simulink library "fsw_lib"  (R2016b)
settings: Solver=VariableStepAuto  StartTime=0.0  StopTime=10.0  RelTol=1e-3
libraries: actuator_processing x1, attitude_estimation_lib x1, command_generation x1, env_estimation_lib x1, mode_selection x1, target_generation_lib x1, telemetry x1
settings Model: Creator=taylorreynolds  LastModifiedBy=Taylor

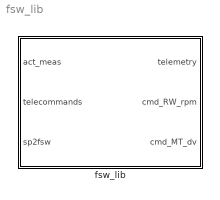
== system fsw_lib ==
  fsw_lib : Subsystem

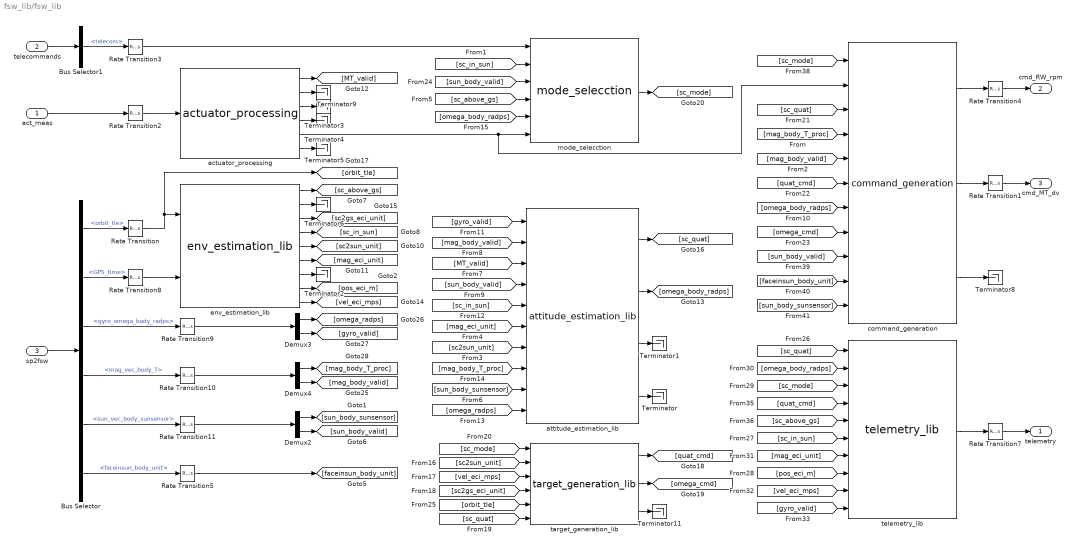
== system fsw_lib/fsw_lib ==
  act_meas : Inport
  telecommands : Inport  Port=2  OutDataTypeStr=Bus: telecommands
  sp2fsw : Inport  Port=3  OutDataTypeStr=Bus: sp2fsw
  Bus Selector : BusSelector  OutputSignals=orbit_tle,GPS_time,gyro_omega_body_radps,mag_vec_body_T,sun_vec_body_sunsensor,faceinsun_body_unit
  Bus Selector1 : BusSelector  OutputSignals=telecom
  Demux2 : Demux  Outputs=[3 1]
  Demux3 : Demux  Outputs=[3 1]
  Demux4 : Demux  Outputs=[3 1]
  Rate Transition : RateTransition  X0=fsw_params.env_estimation.ic.orbit_tle  OutPortSampleTime=fsw_params.sample_time_s
  Rate Transition1 : RateTransition
  Rate Transition{2..3,5,9..11} (6 alike) : RateTransition  OutPortSampleTime=fsw_params.sample_time_s
  Rate Transition4 : RateTransition
  Rate Transition7 : RateTransition
  Rate Transition8 : RateTransition  X0=fsw_params.sensor_processing.gps.ic.time  OutPortSampleTime=fsw_params.sample_time_s
  Terminator{,1..6,8..9,11} (10 alike) : Terminator
  actuator_processing : actuator_processing/actuator_processing
  attitude_estimation_lib : attitude_estimation_lib/attitude_estimation_lib
  command_generation : command_generation/command_generation
  env_estimation_lib : env_estimation_lib/env_estimation_lib
  mode_selecction : mode_selection/mode_selecction
  target_generation_lib : target_generation_lib/target_generation_lib
  telemetry_lib : telemetry/telemetry_lib
  "telemetry " : Outport
  cmd_RW_rpm : Outport  Port=2
  cmd_MT_dv : Outport  Port=3
  wires:
  [sc_above_gs] -> telemetry_lib/5
  Rate Transition5/1 -> [faceinsun_body_unit]
  Bus Selector/6 -> Rate Transition5/1  "<faceinsun_body_unit>"
  [sun_body_valid] -> mode_selecction/3
  [sc_above_gs] -> mode_selecction/4
  [omega_body_radps] -> mode_selecction/5
  actuator_processing/6 -> Terminator5/1
  Rate Transition4/1 -> cmd_RW_rpm/1
  Rate Transition1/1 -> cmd_MT_dv/1
  env_estimation_lib/8 -> [pos_eci_m]
  env_estimation_lib/9 -> [vel_eci_mps]
  [pos_eci_m] -> telemetry_lib/8
  [gyro_valid] -> telemetry_lib/10
  [vel_eci_mps] -> telemetry_lib/9
  [mag_eci_unit] -> telemetry_lib/7
  [sc_in_sun] -> telemetry_lib/6
  [quat_cmd] -> telemetry_lib/4
  [sc_mode] -> telemetry_lib/3
  [omega_body_radps] -> telemetry_lib/2
  [sc_quat] -> telemetry_lib/1
  Rate Transition9/1 -> Demux3/1
  Rate Transition10/1 -> Demux4/1
  Demux4/2 -> [mag_body_valid]
  Demux4/1 -> [mag_body_T_proc]
  Demux3/2 -> [gyro_valid]
  Demux3/1 -> [omega_radps]
  command_generation/2 -> Rate Transition1/1
  [sc_mode] -> command_generation/1
  [sc_mode] -> target_generation_lib/1
  mode_selecction/1 -> [sc_mode]
  target_generation_lib/3 -> Terminator11/1
  Rate Transition3/1 -> mode_selecction/1
  Rate Transition7/1 -> "telemetry "/1
  telecommands/1 -> Bus Selector1/1
  Rate Transition2/1 -> actuator_processing/1
  sp2fsw/1 -> Bus Selector/1
  telemetry_lib/1 -> Rate Transition7/1
  target_generation_lib/2 -> [omega_cmd]
  target_generation_lib/1 -> [quat_cmd]
  [orbit_tle] -> target_generation_lib/5
  [sc_quat] -> target_generation_lib/6
  [sc2gs_eci_unit] -> target_generation_lib/4
  [vel_eci_mps] -> target_generation_lib/3
  [sc2sun_unit] -> target_generation_lib/2
  actuator_processing/5 -> mode_selecction/6, command_generation/2
  attitude_estimation_lib/2 -> [omega_body_radps]
  Bus Selector/2 -> Rate Transition8/1  "<GPS_time>"
  actuator_processing/2 -> Terminator9/1
  actuator_processing/1 -> [MT_valid]
  act_meas/1 -> Rate Transition2/1
  Demux2/2 -> [sun_body_valid]
  Demux2/1 -> [sun_body_sunsensor]
  Bus Selector/5 -> Rate Transition11/1  "<sun_vec_body_sunsensor>"
  Bus Selector/4 -> Rate Transition10/1  "<mag_vec_body_T>"
  Bus Selector/3 -> Rate Transition9/1  "<gyro_omega_body_radps>"
  [sc_in_sun] -> mode_selecction/2
  [mag_body_valid] -> attitude_estimation_lib/2
  [gyro_valid] -> attitude_estimation_lib/1
  env_estimation_lib/4 -> [sc_in_sun]
  [MT_valid] -> attitude_estimation_lib/3
  [sun_body_valid] -> attitude_estimation_lib/4
  [sc_in_sun] -> attitude_estimation_lib/5
  attitude_estimation_lib/4 -> Terminator/1
  attitude_estimation_lib/3 -> Terminator1/1
  env_estimation_lib/5 -> [sc2sun_unit]
  env_estimation_lib/6 -> [mag_eci_unit]
  env_estimation_lib/7 -> Terminator2/1
  actuator_processing/3 -> Terminator3/1
  actuator_processing/4 -> Terminator4/1
  env_estimation_lib/2 -> Terminator6/1
  env_estimation_lib/3 -> [sc2gs_eci_unit]
  [omega_radps] -> attitude_estimation_lib/10
  [sun_body_sunsensor] -> attitude_estimation_lib/9
  [mag_body_T_proc] -> attitude_estimation_lib/8
  [mag_eci_unit] -> attitude_estimation_lib/6
  [sc2sun_unit] -> attitude_estimation_lib/7
  command_generation/1 -> Rate Transition4/1
  command_generation/3 -> Terminator8/1
  attitude_estimation_lib/1 -> [sc_quat]
  env_estimation_lib/1 -> [sc_above_gs]
  Bus Selector/1 -> Rate Transition/1  "<orbit_tle>"
  Rate Transition/1 -> env_estimation_lib/1, [orbit_tle]
  Rate Transition8/1 -> env_estimation_lib/2
  Rate Transition11/1 -> Demux2/1
  Bus Selector1/1 -> Rate Transition3/1  "<telecom>"
  [mag_body_T_proc] -> command_generation/4
  [sc_quat] -> command_generation/3
  [mag_body_valid] -> command_generation/5
  [quat_cmd] -> command_generation/6
  [omega_body_radps] -> command_generation/7
  [omega_cmd] -> command_generation/8
  [sun_body_valid] -> command_generation/9
  [faceinsun_body_unit] -> command_generation/10
  [sun_body_sunsensor] -> command_generation/11
